simulink model "mtask1"  (R2020a)
settings: Solver=VariableStepAuto  StartTime=0.0  StopTime=10.0  RelTol=1e-3
model workspace (MAT data in the model file):
  k = 1
settings Model: Creator=Jesus  LastModifiedBy=root

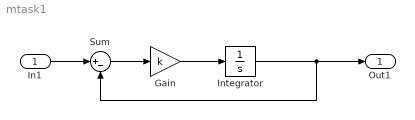
== system mtask1 ==
  In1 : Inport
  Gain : Gain  Gain=k
  Integrator : Integrator
  Sum : Sum  Inputs=|+-
  Out1 : Outport
  wires:
  Gain/1 -> Integrator/1
  Integrator/1 -> Sum/2, Out1/1
  Sum/1 -> Gain/1
  In1/1 -> Sum/1
